simulink library "INT_InjCrv_PiISet"  (R2016b)
settings: Solver=VariableStepAuto  StartTime=0.0  StopTime=10.0  RelTol=1e-3
settings Model: Creator=Administrator  LastModifiedBy=Administrator

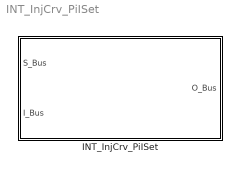
== system INT_InjCrv_PiISet ==
  INT_InjCrv_PiISet : Subsystem

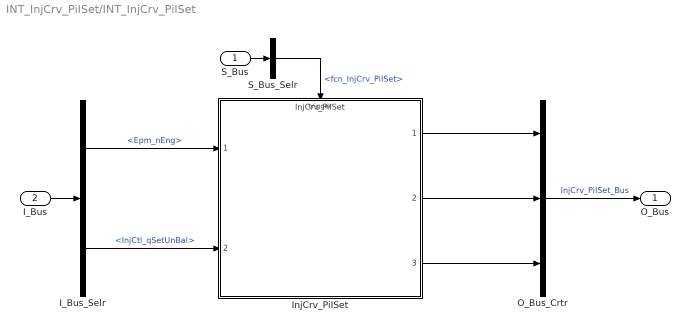
== system INT_InjCrv_PiISet/INT_InjCrv_PiISet ==
  S_Bus : Inport
  I_Bus : Inport  Port=2
  I_Bus_Selr : BusSelector  OutputSignals=Epm_nEng,InjCtl_qSetUnBal
  InjCrv_PiISet : ModelReference  ModelNameDialog=InjCrv_PiISet  SimulationMode=Normal  ModelReferenceVersion=1.12  TriggerPortName=function  TriggerPortTriggerType=function-call  TriggerPortStatesWhenEnabling=held
  O_Bus_Crtr : BusCreator  Inputs=3
  S_Bus_Selr : BusSelector  OutputSignals=fcn_InjCrv_PiISet
  O_Bus : Outport
  wires:
  S_Bus_Selr/1 -> InjCrv_PiISet/Trigger  "<fcn_InjCrv_PiISet>"
  S_Bus/1 -> S_Bus_Selr/1
  I_Bus/1 -> I_Bus_Selr/1
  I_Bus_Selr/1 -> InjCrv_PiISet/1  "<Epm_nEng>"
  I_Bus_Selr/2 -> InjCrv_PiISet/2  "<InjCtl_qSetUnBal>"
  O_Bus_Crtr/1 -> O_Bus/1  "InjCrv_PiISet_Bus"
  InjCrv_PiISet/1 -> O_Bus_Crtr/1
  InjCrv_PiISet/2 -> O_Bus_Crtr/2
  InjCrv_PiISet/3 -> O_Bus_Crtr/3
